simulink model "quarter_sus_win"  (R2025a)
settings: Solver=FixedStepAuto  StartTime=0.0  StopTime=20  FixedStep=0.001  RelTol=1e-3
model workspace (MAT data in the model file):
  Cs : Simulink.Parameter (value not decoded)
  Cy_f1 = 128915.5
  Cy_r1 = 85943.6
  G0 : Simulink.Parameter (value not decoded)
  IDA_ISD_PBC_bd : Simulink.Parameter (value not decoded)
  IDA_ISD_PBC_c1 : Simulink.Parameter (value not decoded)
  IDA_ISD_PBC_k1 : Simulink.Parameter (value not decoded)
  IDA_ISD_PBC_k2 : Simulink.Parameter (value not decoded)
  IDA_ISD_PBC_r1 : Simulink.Parameter (value not decoded)
  IDA_PBC_cd4 = 2000
  IDA_PBC_kd2 = 10000
  IDA_PBC_r1 = 1.5
  IDA_PBC_r2 = 0.44
  ISD_1_b : Simulink.Parameter (value not decoded)
  ISD_1_c : Simulink.Parameter (value not decoded)
  ISD_1_k1 : Simulink.Parameter (value not decoded)
  ISD_1_k2 : Simulink.Parameter (value not decoded)
  Izz1 = 1536.7
  Ks : Simulink.Parameter (value not decoded)
  Kt : Simulink.Parameter (value not decoded)
  Q : Simulink.Parameter (value not decoded)
  Q_F : Simulink.Parameter (value not decoded)
  Q_b_deflec : Simulink.Parameter (value not decoded)
  Q_dot : Simulink.Parameter (value not decoded)
  Q_dot_s : Simulink.Parameter (value not decoded)
  Q_dot_s_h : Simulink.Parameter (value not decoded)
  Q_dot_u : Simulink.Parameter (value not decoded)
  Q_flec : Simulink.Parameter (value not decoded)
  Q_flec_t : Simulink.Parameter (value not decoded)
  SHADD_alpha : Simulink.Parameter (value not decoded)
  a1 = 1.015
  a_max : Simulink.Parameter (value not decoded)
  a_min : Simulink.Parameter (value not decoded)
  adva_max : Simulink.Parameter (value not decoded)
  adva_min : Simulink.Parameter (value not decoded)
  as_max : Simulink.Parameter (value not decoded)
  b1 = 1.895
  b_deflec : Simulink.Parameter (value not decoded)
  bump_height : Simulink.Parameter (value not decoded)
  bump_lenth : Simulink.Parameter (value not decoded)
  bump_start : Simulink.Parameter (value not decoded)
  damper_param : Simulink.Parameter (value not decoded)
  deflec_max : Simulink.Parameter (value not decoded)
  done_range : Simulink.Parameter (value not decoded)
  f0 : Simulink.Parameter (value not decoded)
  h1 = 0.54
  imp_Cs : Simulink.Parameter (value not decoded)
  imp_Ks : Simulink.Parameter (value not decoded)
  imp_Ms : Simulink.Parameter (value not decoded)
  inerter_b : Simulink.Parameter (value not decoded)
  inerter_b_2 : Simulink.Parameter (value not decoded)
  inerter_c : Simulink.Parameter (value not decoded)
  inerter_k : Simulink.Parameter (value not decoded)
  inerter_k_2 : Simulink.Parameter (value not decoded)
  ms : Simulink.Parameter (value not decoded)
  mu : Simulink.Parameter (value not decoded)
  noise_seed : Simulink.Parameter (value not decoded)
  omega_1 : Simulink.Parameter (value not decoded)
  omega_2 : Simulink.Parameter (value not decoded)
  omega_3 : Simulink.Parameter (value not decoded)
  omega_4 : Simulink.Parameter (value not decoded)
  punish_Q : Simulink.Parameter (value not decoded)
  punish_R : Simulink.Parameter (value not decoded)
  reward_w_as : Simulink.Parameter (value not decoded)
  reward_w_au : Simulink.Parameter (value not decoded)
  reward_w_defv : Simulink.Parameter (value not decoded)
  road_seed : Simulink.Parameter (value not decoded)
  road_type : Simulink.Parameter (value not decoded)
  sigma_f1 = 0.1
  sigma_r1 = 0.1
  sine_amp : Simulink.Parameter (value not decoded)
  sine_freq : Simulink.Parameter (value not decoded)
  u : Simulink.Parameter (value not decoded)
  vs0 : Simulink.Parameter (value not decoded)
  vu0 : Simulink.Parameter (value not decoded)
  x_max : Simulink.Parameter (value not decoded)
  x_min : Simulink.Parameter (value not decoded)
  xs0 : Simulink.Parameter (value not decoded)
  xu0 : Simulink.Parameter (value not decoded)
symbols that are objects in the model workspace (value not decoded): a_max, a_min, b_deflec, bump_height, bump_lenth, bump_start, Cs, damper_param, f0, G0, IDA_ISD_PBC_bd, IDA_ISD_PBC_c1, IDA_ISD_PBC_k1, IDA_ISD_PBC_k2, IDA_ISD_PBC_r1, imp_Cs, imp_Ks, imp_Ms, Ks, Kt, ms, mu, omega_1, omega_2, omega_3, omega_4, Q_b_deflec, Q_dot_s, Q_dot_s_h, Q_dot_u, Q_F, Q_flec, Q_flec_t, road_type, SHADD_alpha, sine_amp, sine_freq, vs0, vu0, xs0, xu0
undefined symbols (not defined in the file or in its folder): ADD, Force, IDA, Imp, PBC, SH, Train, Validation
libraries: fl_lib x32, nesl_utility x27, sdl_lib x2, deeplib x1, simulink x1
(part 3 of 6)

== system quarter_sus_win/QuarterSuspension /road_profile/Subsystem ==
  1-D Lookup Table : Lookup_n-D  NumberOfTableDimensions=1  BreakpointsSpecification=Even spacing  BreakpointsForDimension1Source=Input port  BreakpointsForDimension1=[-5:5]  BreakpointsForDimension1FirstPoint=0  BreakpointsForDimension1Spacing=0.001  IndexSearchMethod=Evenly spaced points  BeginIndexSearchUsingPreviousIndexResult=on  TableSource=Input port  Table=tanh([-5:5])  InternalRulePriority=Speed  RndMeth=Simplest
      settings: InputPortMap=u0,p221
  Add : Sum
  Clock : Clock
  Gain2 : Gain  Gain=-2*pi*f0
  gp_sample : Constant  Value=[0.170025278484339 0.175816136620074 0.181473484521814 0.187074816885986 0.192577523447574 0.197954331997763 0.203244446980971 0.208440378667596 0.21359007870523 0.218630897005782 0.223526682119238 0.228421308448727 0.233179765964321 0.237855612427958 0.242464189623578 0.246973678945713 0.251407769980235 0.255786282349279 0.260080773520862 0.264305172612954 0.268450087721149 0.272504068303003 0.276527112378618 0.28048558268508 0.284361508143581 0.288192952337151 0.291959936182145 0.295659830212886 0.2993206542816 0.302910781523847 0.306480729123347 0.309964753616006 0.313415988099253 0.316824203215788 0.320156693859928 0.323518500764006 0.326797753070224 0.330033937407187 0.333270889875012 0.33642016818152 0.339579796548874 0.342696396101878 0.345793758734641 0.348861872560406 0.351891086031793 0.354916811622082 0.357914072447518 0.360903897082363 0.363877974875121 0.366835387249315 0.369754982846105 0.372688864801886 0.375588395993681 0.378488059766184 0.381392014403952 0.384301422864585 0.387165931517105 0.390057795053213 0.392930994550214 0.395824508581227 0.398680028812144 0.401565976917868 0.404451752871203 0.407343972172829 0.410242837920754 0.413125982866568 0.416005338904083 0.418910600377238 0.421811478304582 0.424764495207341 0.427663395468628 0.430610127207448 0.433543666967063 0.436507096921314 0.439451263091937 0.442408633179025 0.445378412057655 0.448380374652938 0.451368696576693 0.454370858165168 0.45740260717743 0.460417951439973 0.463450043741481 0.46650952238807 0.469537860198321 0.472611195603313 0.475683148473323 0.478748557197063 0.481834839370814 0.484906408990426 0.487993160586329 0.491099115664871 0.494207158371036 0.497338162652649 0.500418728584987 0.503536796359788 0.506645952707285 0.509733679856585 0.512851682787171 0.515937955244445 0.51906276090946 0.522141069096423 0.525238595359704 0.528313056100158 0.53139422842638 0.534447795549369 0.53751047671874 0.540555684438933 0.543598184556746 0.546595802352358 0.549567576961909 0.552551008963177 0.555531350622218 0.558444181371885 0.561378290919564 0.564262781138414 0.567145180736086 0.569949093946312 0.572771716686528 0.575537321693657 0.578329736250285 0.58103314888404 0.583726486831957 0.586350389375156 0.588962636645158 0.591533227993985 0.594078691045764 0.596555127806964 0.599011117119705 0.601380604746945 0.603744784318164 0.606041110867711 0.608281267208009 0.610500691450385 0.612648353332122 0.614740792984746 0.616762553266001 0.618767592897855 0.620685857117294 0.622542818240381 0.624347616116886 0.626083890011176 0.627739909529867 0.629359301630112 0.630893369686012 0.632361352405345 0.633758216516723 0.635092657627579 0.63633149639614 0.637544038338831 0.638653850584212 0.639685659927166 0.640645214050705 0.641517903975367 0.642340077645861 0.64305482957042 0.643691081367558 0.644275704665605 0.644743238461787 0.64513571313418 0.645450405862105 0.645670891009415 0.645806140690156 0.645901563808983 0.645872361975845 0.645747666982458 0.645526884426396 0.645234005665105 0.644856726061085 0.644396217971618 0.643812320253848 0.643141452075983 0.642396339334973 0.641573260399067 0.64064477278748 0.639624574014781 0.63850450289799 0.637300083903877 0.63599210380528 0.634612376797282 0.633101757083729 0.631536861318424 0.629847956181882 0.628081468339218 0.626227728044514 0.624279575789236 0.622208107109269 0.620088917289921 0.617850794869455 0.615515930762129 0.613092345418776 0.61057657015653 0.607967173999525 0.605269925369424 0.602478392704001 0.599604584814701 0.596642683413984 0.593572669001915 0.590413107246599 0.587179490960088 0.583845103047985 0.580410906090815 0.576922051950385 0.573322709321438 0.569640003160408 0.565877500553624 0.562023982255742 0.558073388456057 0.554057539366014 0.549952397006264 0.545759966756969 0.541516079847749 0.537143653587366 0.532716409732544 0.528204007330299 0.523609248553631 0.518952296934778 0.514210092289194 0.509415423296786 0.504511486766229 0.499538770137798 0.494532714110356 0.48943111929704 ...(+555678 chars)]
  gp_t : Constant  Value=[0;0.00100003333444448;0.00200006666888896;0.00300010000333344;0.00400013333777793;0.00500016667222241;0.00600020000666689;0.00700023334111137;0.00800026667555585;0.00900030001000033;0.0100003333444448;0.0110003666788893;0.0120004000133338;0.0130004333477783;0.0140004666822227;0.0150005000166672;0.0160005333511117;0.0170005666855562;0.0180006000200007;0.0190006333544451;0.0200006666888896;0.0210007000233341;0.0220007333577786;0.0230007666922231;0.0240008000266676;0.025000833361112;0.0260008666955565;0.027000900030001;0.0280009333644455;0.02900096669889;0.0300010000333344;0.0310010333677789;0.0320010667022234;0.0330011000366679;0.0340011333711124;0.0350011667055568;0.0360012000400013;0.0370012333744458;0.0380012667088903;0.0390013000433348;0.0400013333777793;0.0410013667122237;0.0420014000466682;0.0430014333811127;0.0440014667155572;0.0450015000500017;0.0460015333844461;0.0470015667188906;0.0480016000533351;0.0490016333877796;0.0500016667222241;0.0510017000566686;0.052001733391113;0.0530017667255575;0.054001800060002;0.0550018333944465;0.056001866728891;0.0570019000633354;0.0580019333977799;0.0590019667322244;0.0600020000666689;0.0610020334011134;0.0620020667355579;0.0630021000700023;0.0640021334044468;0.0650021667388913;0.0660022000733358;0.0670022334077803;0.0680022667422247;0.0690023000766692;0.0700023334111137;0.0710023667455582;0.0720024000800027;0.0730024334144471;0.0740024667488916;0.0750025000833361;0.0760025334177806;0.0770025667522251;0.0780026000866696;0.079002633421114;0.0800026667555585;0.081002700090003;0.0820027334244475;0.083002766758892;0.0840028000933364;0.0850028334277809;0.0860028667622254;0.0870029000966699;0.0880029334311144;0.0890029667655589;0.0900030001000033;0.0910030334344478;0.0920030667688923;0.0930031001033368;0.0940031334377813;0.0950031667722257;0.0960032001066702;0.0970032334411147;0.0980032667755592;0.0990033001100037;0.100003333444448;0.101003366778893;0.102003400113337;0.103003433447782;0.104003466782226;0.105003500116671;0.106003533451115;0.10700356678556;0.108003600120004;0.109003633454448;0.110003666788893;0.111003700123337;0.112003733457782;0.113003766792226;0.114003800126671;0.115003833461115;0.11600386679556;0.117003900130004;0.118003933464449;0.119003966798893;0.120004000133338;0.121004033467782;0.122004066802227;0.123004100136671;0.124004133471116;0.12500416680556;0.126004200140005;0.127004233474449;0.128004266808894;0.129004300143338;0.130004333477783;0.131004366812227;0.132004400146672;0.133004433481116;0.134004466815561;0.135004500150005;0.136004533484449;0.137004566818894;0.138004600153338;0.139004633487783;0.140004666822227;0.141004700156672;0.142004733491116;0.143004766825561;0.144004800160005;0.14500483349445;0.146004866828894;0.147004900163339;0.148004933497783;0.149004966832228;0.150005000166672;0.151005033501117;0.152005066835561;0.153005100170006;0.15400513350445;0.155005166838895;0.156005200173339;0.157005233507784;0.158005266842228;0.159005300176673;0.160005333511117;0.161005366845562;0.162005400180006;0.16300543351445;0.164005466848895;0.165005500183339;0.166005533517784;0.167005566852228;0.168005600186673;0.169005633521117;0.170005666855562;0.171005700190006;0.172005733524451;0.173005766858895;0.17400580019334;0.175005833527784;0.176005866862229;0.177005900196673;0.178005933531118;0.179005966865562;0.180006000200007;0.181006033534451;0.182006066868896;0.18300610020334;0.184006133537785;0.185006166872229;0.186006200206674;0.187006233541118;0.188006266875563;0.189006300210007;0.190006333544451;0.191006366878896;0.19200640021334;0.193006433547785;0.194006466882229;0.195006500216674;0.196006533551118;0.197006566885563;0.198006600220007;0.199006633554452;0.200006666888896;0.201006700223341;0.202006733557785;0.20300676689223;0.204006800226674;0.205006833561119;0.206006866895563;0.207006900230008;0.208006933564452;0.209006966898897;0.210007000233341;0.211007033567786;0.21200706690223;0.213007100236675;0.214007133571119;0.215007166905564;0.216007200240008;0.217007233574452 ...(+503836 chars)]
  xr : Integrator
  "Road " : Outport
  wires:
  gp_t/1 -> ?
  Clock/1 -> 1-D Lookup Table/1
  gp_sample/1 -> 1-D Lookup Table/2
  Gain2/1 -> Add/2
  xr/1 -> "Road "/1, Gain2/1
  Add/1 -> xr/1
  1-D Lookup Table/1 -> Add/1
